simulink library "IEEE80211a_lib"  (Simulink 5.0)
libraries: commblkintrlv2 x4, commdigbbndam2 x3, commsequence2 x2, commcnvcod2 x2, commutil2 x1, dspsigops x1, simulink x1
settings Model: Creator=y  LastModifiedBy=Owner

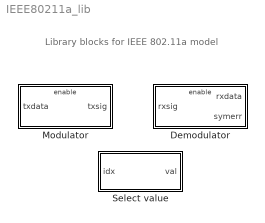
== system IEEE80211a_lib ==
  note: Library blocks for IEEE 802.11a model
  Demodulator : Subsystem  mask(QAM Demodulator-Decoder.){numSymbols=960, modulation=BPSK, code=3/4, trellisStructure=poly2trellis(7, [171 133]), punctureVector=[1 1 1 0 0 1].', vtbd=34}
      mask prompts: numSymbols "Number of symbols per frame:"; trellisStructure "Trellis:"; punctureVector "Puncture vector:"; vtbd "Viterbi trace back depth:"
      mask help: Demodulator has option to zero-pad output, so that a bank of different modulators can share the same output frame size.
      mask init:
      | % number of bits per symbol
      | switch modulation
      | 	case 'BPSK', Nb1 = 1;
      | 	case 'QPSK', Nb1 = 2;
      | 	case '16-QAM', Nb1 = 4;
      | 	case '64-QAM', Nb1 = 6;
      | end
      | 
      | modOrder = 2.^Nb1;
      | Nb = numSymbols * Nb1; % tx bits per block
      | codeRate = str2num(strvcat(code)).';
      | bitsPerBlock = Nb .* codeRate;
      | 
      | % interleaver
      | interleaverRows = 16;
      | if rem(Nb, interleaverRows)
      | 	error('Number of transmitted bits per block must be multiple of 16.')
      | end
      | interleaverCols = Nb / interleaverRows;
      | interleaverElements = [...
      |             2*floor( [0:Nb-1]/2 ) + ...
      |             mod( ([0:Nb-1] + Nb - floor( interleaverRows*[0:Nb-1]/Nb ) ), 2 ) ...
      |             + 1]';
      mask Display:
      | disp(['Demodulator\n' modulation ' ' code])
      | port_label('input', 1, ' ')
      | port_label('output', 1, ' ')
      | port_label('output', 2, 'err')
  Modulator : Subsystem  mask(QAM Modulator-Coder.){numSymbols=960, modulation=BPSK, code=3/4, trellisStructure=poly2trellis(7, [171 133]), punctureVector=[1 1 1 0 0 1].'}
      mask prompts: numSymbols "Number of symbols per frame:"; trellisStructure "Trellis:"; punctureVector "Puncture vector:"
      mask help: Modulator gates incoming bits so that a bank of different modulators can share the same input frame size.
      mask init: same as IEEE80211a_lib/Demodulator
      mask Display: disp(['Modulator\n' modulation ' ' code])
  Select value : Subsystem  mask{vector=[0 1 2]}
      mask help: Using MATLAB-style indexing, output value of selected element of vector.
      mask Display: disp('Select\nValue')

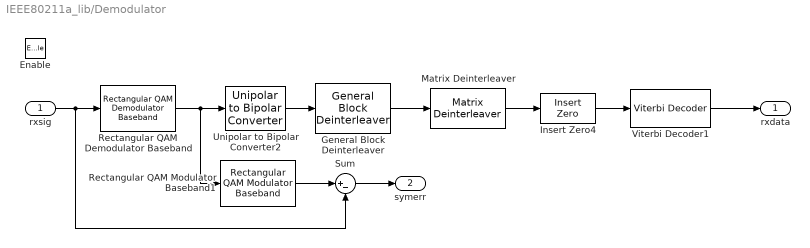
== system IEEE80211a_lib/Demodulator ==
  rxsig : Inport
  Enable : EnablePort
  General Block Deinterleaver : commblkintrlv2/General Block Deinterleaver  elements=interleaverElements
  Insert Zero4 : commsequence2/Insert Zero  insertZeroVector=punctureVector
  Matrix Deinterleaver : commblkintrlv2/Matrix Deinterleaver  Nrows=interleaverRows  Ncols=interleaverCols
  Rectangular QAM Demodulator Baseband : commdigbbndam2/Rectangular QAM Demodulator Baseband  M=modOrder  OutType=Bit  Dec=Gray  PowType=Average Power  MinDist=2  AvgPow=1  PeakPow=1  Ph=0  numSamp=1
  Rectangular QAM Modulator Baseband1 : commdigbbndam2/Rectangular QAM Modulator Baseband  M=modOrder  InType=Bit  Enc=Gray  PowType=Average Power  MinDist=2  AvgPow=1  PeakPow=1  Ph=0  numSamp=1
  Sum : Sum  Inputs=|+-  SaturateOnIntegerOverflow=on
  Unipolar to Bipolar Converter2 : commutil2/Unipolar to Bipolar Converter  M=2  polarity=Negative
  Viterbi Decoder1 : commcnvcod2/Viterbi Decoder  trellis=trellisStructure  dectype=Unquantized  nsdecb=4  tbdepth=vtbd  opmode=Continuous  reset=off
  rxdata : Outport  OutputWhenDisabled=reset  InitialOutput=0
  symerr : Outport  Port=2  OutputWhenDisabled=reset  InitialOutput=0
  wires:
  Rectangular QAM Demodulator Baseband/1 -> Unipolar to Bipolar Converter2/1, Rectangular QAM Modulator Baseband1/1
  Insert Zero4/1 -> Viterbi Decoder1/1
  rxsig/1 -> Rectangular QAM Demodulator Baseband/1, Sum/2
  Unipolar to Bipolar Converter2/1 -> General Block Deinterleaver/1
  Viterbi Decoder1/1 -> rxdata/1
  Rectangular QAM Modulator Baseband1/1 -> Sum/1
  Sum/1 -> symerr/1
  Matrix Deinterleaver/1 -> Insert Zero4/1
  General Block Deinterleaver/1 -> Matrix Deinterleaver/1

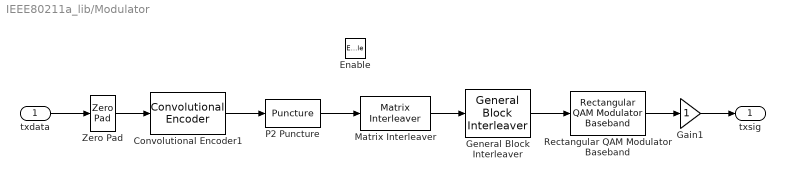
== system IEEE80211a_lib/Modulator ==
  txdata : Inport
  Enable : EnablePort
  Convolutional Encoder1 : commcnvcod2/Convolutional Encoder  trellis=trellisStructure  reset=None
  Gain1 : Gain  SaturateOnIntegerOverflow=on
  General Block Interleaver : commblkintrlv2/General Block Interleaver  elements=interleaverElements
  Matrix Interleaver : commblkintrlv2/Matrix Interleaver  Nrows=interleaverRows  Ncols=interleaverCols
  P2 Puncture : commsequence2/Puncture  punctureVector=punctureVector
  Rectangular QAM Modulator Baseband : commdigbbndam2/Rectangular QAM Modulator Baseband  M=modOrder  InType=Bit  Enc=Gray  PowType=Average Power  MinDist=2  AvgPow=1  PeakPow=1  Ph=0  numSamp=1
  Zero Pad : dspsigops/Zero Pad  padSigAt=End  zpadAlong=Columns  padNumOutRowsSpecMethod=User-specified  numOutRows=bitsPerBlock  padNumOutColsSpecMethod=User-specified  numOutCols=1  trunc_flag=None
      settings: AttributesFormatString=\n
  txsig : Outport
  wires:
  General Block Interleaver/1 -> Rectangular QAM Modulator Baseband/1
  P2 Puncture/1 -> Matrix Interleaver/1
  Matrix Interleaver/1 -> General Block Interleaver/1
  Convolutional Encoder1/1 -> P2 Puncture/1
  Zero Pad/1 -> Convolutional Encoder1/1
  txdata/1 -> Zero Pad/1
  Gain1/1 -> txsig/1
  Rectangular QAM Modulator Baseband/1 -> Gain1/1

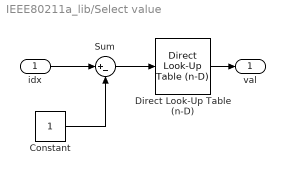
== system IEEE80211a_lib/Select value ==
  idx : Inport
  Constant : Constant
  Direct Look-Up Table (n-D) : simulink/Look-Up Tables/Direct Look-Up Table (n-D)  maskTabDims=1  explicitNumDims=1  outDims=Element  tabIsInput=off  mxTable=vector  clipFlag=Warning
  Sum : Sum  Inputs=|+-  SaturateOnIntegerOverflow=on
  val : Outport
  wires:
  Constant/1 -> Sum/2
  Sum/1 -> Direct Look-Up Table (n-D)/1
  Direct Look-Up Table (n-D)/1 -> val/1
  idx/1 -> Sum/1
